simulink model "sampleModel2072_pp"  (R2021a)
settings: Solver=VariableStepAuto  StartTime=0.0  StopTime=10.0  RelTol=1e-3
undefined symbols (not defined in the file or in its folder): DiscIntNeverNeededParam, magnitude, Newton, Raphson
libraries: simulink x184, pid_lib x33
(part 3 of 5)

== system sampleModel2072_pp/cfblk39/cfblk6 ==
  cfblk1 : Inport
  cfblk10 : Signum
  cfblk11 : Sin  TimeSource=Use external signal  SampleTime=0
  cfblk12 : Product  Inputs=**
  cfblk13 : Product
  cfblk14 : Delay  SampleTime=1
  cfblk3 : pid_lib/PID Controller  Controller=PID  Form=Parallel  TimeDomain=Discrete-time  UseExternalTs=off  SampleTime=1  IntegratorMethod=Forward Euler  FilterMethod=Forward Euler  ControllerParametersSource=internal  P=1  I=1  D=0  UseFilter=on  N=100  TunerSelectOption=Transfer Function Based (PID Tuner App)  InitialConditionSource=internal  InitialConditionForIntegrator=0  InitialConditionForFilter=0  DifferentiatorICPrevScaledInput=0  ExternalReset=none  TrackingMode=off  Kt=1  LimitOutput=off  SatLimitsSource=internal  UpperSaturationLimit=inf  LowerSaturationLimit=-inf  LinearizeAsGain=off  AntiWindupMode=none  Kb=1  POutMin=[]  POutMax=[]  IOutMin=[]  IOutMax=[]  DOutMin=[]  DOutMax=[]  NOutMin=[]  NOutMax=[]  SumOutMin=[]  SumOutMax=[]  SaturationOutMin=[]  SaturationOutMax=[]  PParamMin=[]  PParamMax=[]  IParamMin=[]  IParamMax=[]  DParamMin=[]  DParamMax=[]  NParamMin=[]  NParamMax=[]  KbParamMin=[]  KbParamMax=[]  KtParamMin=[]  KtParamMax=[]  KbOutMin=[]  KbOutMax=[]  KtOutMin=[]  KtOutMax=[]  IntegratorOutMin=[]  IntegratorOutMax=[]  FilterOutMin=[]  FilterOutMax=[]  SumI1OutMin=[]  SumI1OutMax=[]  SumI2OutMin=[]  SumI2OutMax=[]  SumI3OutMin=[]  SumI3OutMax=[]  SumI4OutMin=[]  SumI4OutMax=[]  SumDOutMin=[]  SumDOutMax=[]  DifferentiatorOutMin=[]  DifferentiatorOutMax=[]  FilterDiffOutCoefMin=[]  FilterDiffOutCoefMax=[]  ReciprocalOutMin=[]  ReciprocalOutMax=[]  SumDenOutMin=[]  SumDenOutMax=[]  SumNumOutMin=[]  SumNumOutMax=[]  DivideOutMin=[]  DivideOutMax=[]  UdiffTsProdOutMin=[]  UdiffTsProdOutMax=[]  NTsProdOutMin=[]  NTsProdOutMax=[]  UintegralTsProdOutMin=[]  UintegralTsProdOutMax=[]  UngainTsProdOutMin=[]  UngainTsProdOutMax=[]  IntegratorContinuousStateAttributes=''  IntegratorStateMustResolveToSignalObject=off  IntegratorRTWStateStorageClass=Auto  FilterContinuousStateAttributes=''  FilterStateMustResolveToSignalObject=off  FilterRTWStateStorageClass=Auto  ParallelPVariant=InternalParameters  IdealPVariant=Disabled  IVariant=InternalParameters  DVariant=InternalParameters  IntegratorVariant=Discrete  SatVariant=Disabled  AWVariant=Passthrough  PCopyVariant=Disabled  TRVariant=Disabled  FdbkBlocksVariant=Forward  IdealPFdbkVariant=Disabled  SatFdbkVariant=Disabled  DerivativeFilterVariant=ForwardEulerFilter  NVariant=InternalParameters  NCopyVariant=Disabled  FilterICVariant=InternalICsFilter  IntegratorICVariant=InternalICs  ExternalResetVariant=Disabled  TRSumVariant=Passthrough  SumFdbkVariant=Disabled  SumVariant=Sum_PID  TsampFilterVariant=InternalTs  TsampNgainVariant=Passthrough  TsampIntegralVariant=Passthrough  ExternalSaturationOutDataTypeStr=Inherit: Same as second input
  cfblk4 : simulink/Discrete/Transfer Fcn Lead or Lag  PoleZ=0.95  ZeroZ=0.75  ICPrevOutput=0.0  ICPrevInput=0.0  DoSatur=off
      settings: SourceProductBaseCode=SL
  cfblk5 : Product  Inputs=**
  cfblk6 : Sqrt  Operator=rSqrt  AlgorithmType=Newton-Raphson  SaturateOnIntegerOverflow=on
  cfblk7 : Sqrt  SaturateOnIntegerOverflow=on
  cfblk8 : Gain  Gain=[-748975620.675067]
  cfblk9 : Reshape
  cfblk2 : Outport
  wires:
  cfblk5/1 -> cfblk3/1
  cfblk7/1 -> cfblk10/1
  cfblk4/1 -> cfblk7/1
  cfblk3/1 -> cfblk6/1
  cfblk1/1 -> cfblk9/1
  cfblk12/1 -> cfblk11/1
  cfblk10/1 -> cfblk13/1, cfblk12/1
  cfblk6/1 -> cfblk8/1
  cfblk9/1 -> cfblk4/1
  cfblk11/1 -> cfblk2/1
  cfblk13/1 -> cfblk5/1, cfblk5/2, cfblk12/2
  cfblk8/1 -> cfblk14/1
  cfblk14/1 -> cfblk13/2

== system sampleModel2072_pp/cfblk39/cfblk7 ==
  cfblk1 : Inport
  cfblk3 : simulink/Discrete/Transfer Fcn First Order  PoleZ=0.95  ICPrevOutput=0.0  DoSatur=off
  cfblk4 : Sqrt  SaturateOnIntegerOverflow=on
  cfblk5 : Product  Inputs=**
  cfblk6 : Gain  Gain=[-247254324.663936]
  cfblk7 : Sqrt  SaturateOnIntegerOverflow=on
  cfblk8 : Polyval  Coefs=[ +2.081618890e-019, -1.441693666e-014, +4.719686976e-010, -8.536869453e-006, +1.621573104e-001, -8.087801117e+001 ]
  cfblk9 : Delay  SampleTime=1
  cfblk2 : Outport
  wires:
  cfblk3/1 -> cfblk8/1
  cfblk7/1 -> cfblk3/1
  cfblk6/1 -> cfblk4/1
  cfblk4/1 -> cfblk2/1
  cfblk5/1 -> cfblk7/1
  cfblk1/1 -> cfblk6/1, cfblk5/2
  cfblk8/1 -> cfblk9/1
  cfblk9/1 -> cfblk5/1

== system sampleModel2072_pp/cfblk39/cfblk8 ==
  cfblk1 : Inport
  cfblk10 : Gain  Gain=[-609988645.580152]
  cfblk11 : Sqrt  SaturateOnIntegerOverflow=on
  cfblk12 : Rounding
  cfblk13 : Reshape
  cfblk14 : Delay  SampleTime=1
  cfblk15 : Delay  SampleTime=1
  cfblk3 : DiscreteZeroPole  Poles=[0 0.5]  Gain=1
  cfblk4 : DiscreteIntegrator  ICPrevOutput=DiscIntNeverNeededParam  ICPrevScaledInput=DiscIntNeverNeededParam
  cfblk5 : simulink/Discrete/Tapped Delay  vinit=0.0  samptime=-1  NumDelays=1  DelayOrder=Oldest  includeCurrent=off
  cfblk6 : Sum  Inputs=|++
  cfblk7 : Rounding
  cfblk8 : Product
  cfblk9 : Math  Operator=log  SaturateOnIntegerOverflow=on
  cfblk2 : Outport
  wires:
  cfblk8/1 -> cfblk9/1
  cfblk4/1 -> cfblk11/1
  cfblk12/1 -> cfblk2/1, cfblk13/1
  cfblk6/1 -> cfblk3/1
  cfblk3/1 -> cfblk8/1
  cfblk10/1 -> cfblk4/1
  cfblk5/1 -> cfblk6/1
  cfblk11/1 -> cfblk7/1
  cfblk1/1 -> cfblk6/2, cfblk10/1
  cfblk7/1 -> cfblk5/1
  cfblk9/1 -> cfblk14/1
  cfblk14/1 -> cfblk8/2
  cfblk13/1 -> cfblk15/1
  cfblk15/1 -> cfblk12/1

== system sampleModel2072_pp/cfblk40/cfblk10 ==
  cfblk1 : Inport
  cfblk8 : Inport  Port=2
  cfblk3 : simulink/Discrete/Transfer Fcn First Order  PoleZ=0.95  ICPrevOutput=0.0  DoSatur=off
  cfblk4 : simulink/Discrete/Transfer Fcn Lead or Lag  PoleZ=0.95  ZeroZ=0.75  ICPrevOutput=0.0  ICPrevInput=0.0  DoSatur=off
      settings: SourceProductBaseCode=SL
  cfblk5 : Rounding
  cfblk6 : Sum
  cfblk7 : MinMax  Function=max
  cfblk2 : Outport
  wires:
  cfblk7/1 -> cfblk5/1
  cfblk1/1 -> cfblk4/1
  cfblk8/1 -> cfblk7/1
  cfblk4/1 -> cfblk6/1
  cfblk5/1 -> cfblk3/1
  cfblk3/1 -> cfblk6/2
  cfblk6/1 -> cfblk2/1

== system sampleModel2072_pp/cfblk40/cfblk11 ==
  cfblk1 : Inport
  cfblk10 : Sum  Inputs=+-
  cfblk11 : Sqrt  SaturateOnIntegerOverflow=on
  cfblk12 : Abs
  cfblk13 : Sum  Inputs=+
  cfblk14 : Product  Inputs=**
  cfblk15 : MinMax  Function=max  Inputs=3
  cfblk16 : Delay  SampleTime=1
  cfblk17 : Delay  SampleTime=1
  cfblk18 : Delay  SampleTime=1
  cfblk3 : simulink/Discrete/Transfer Fcn Real Zero  ZeroZ=0.75  ICPrevInput=0.0  DoSatur=off
      settings: SourceProductBaseCode=SL
  cfblk4 : MinMax  Function=max  Inputs=2
  cfblk5 : PermuteDimensions
  cfblk6 : Trigonometry
  cfblk7 : Signum
  cfblk8 : Sqrt  SaturateOnIntegerOverflow=on
  cfblk9 : Gain  Gain=[-702374637.657523]
  cfblk2 : Outport
  wires:
  cfblk3/1 -> cfblk8/1
  cfblk6/1 -> cfblk10/1, cfblk7/1
  cfblk13/1 -> cfblk3/1
  cfblk1/1 -> cfblk11/1
  cfblk14/1 -> cfblk15/1
  cfblk12/1 -> cfblk6/1, cfblk15/3, cfblk9/1
  cfblk11/1 -> cfblk4/1, cfblk13/1
  cfblk9/1 -> cfblk15/2, cfblk2/1
  cfblk4/1 -> cfblk10/2
  cfblk5/1 -> cfblk12/1
  cfblk8/1 -> cfblk14/2
  cfblk10/1 -> cfblk16/1
  cfblk16/1 -> cfblk4/2
  cfblk15/1 -> cfblk17/1
  cfblk17/1 -> cfblk14/1
  cfblk7/1 -> cfblk18/1
  cfblk18/1 -> cfblk5/1

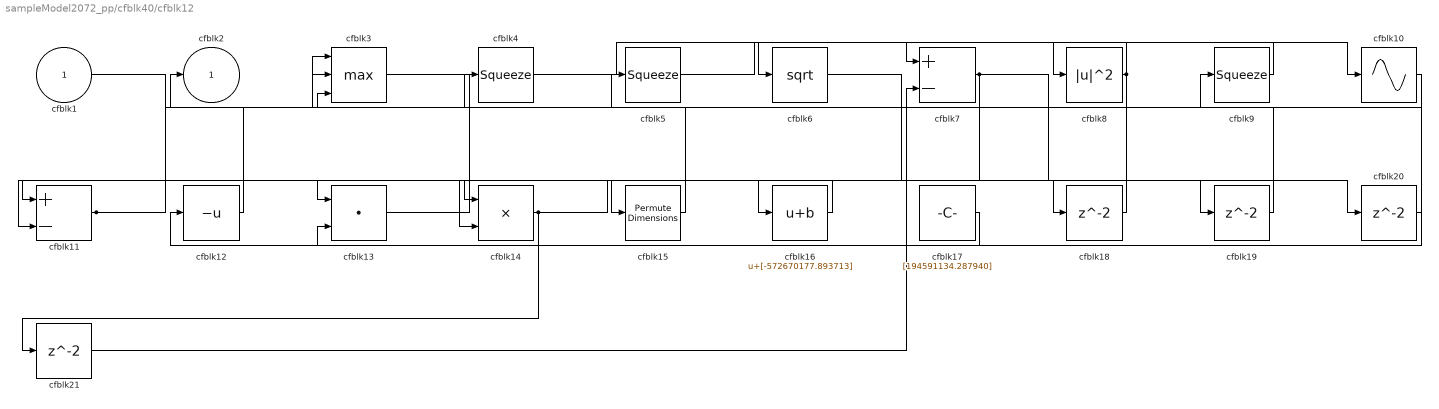
== system sampleModel2072_pp/cfblk40/cfblk12 ==
  cfblk1 : Inport
  cfblk10 : Sin  TimeSource=Use external signal  SampleTime=0
  cfblk11 : Sum  Inputs=+-
  cfblk12 : UnaryMinus
  cfblk13 : DotProduct  InputSameDT=on  OutDataTypeStr=Inherit: Inherit via internal rule
  cfblk14 : Product  Inputs=**
  cfblk15 : PermuteDimensions
  cfblk16 : Bias  Bias=[-572670177.893713]
  cfblk17 : Constant  Value=[194591134.287940]  SampleTime=1
  cfblk{18..21} (4 alike) : Delay  SampleTime=1
  cfblk3 : MinMax  Function=max  Inputs=3
  cfblk4 : Squeeze
  cfblk5 : Squeeze
  cfblk6 : Sqrt  SaturateOnIntegerOverflow=on
  cfblk7 : Sum  Inputs=+-
  cfblk8 : Math  Operator=magnitude^2  SaturateOnIntegerOverflow=on
  cfblk9 : Squeeze
  cfblk2 : Outport
  wires:
  cfblk4/1 -> cfblk10/1
  cfblk3/1 -> cfblk16/1
  cfblk7/1 -> cfblk14/2, cfblk19/1
  cfblk10/1 -> cfblk12/1
  cfblk14/1 -> cfblk20/1, cfblk21/1
  cfblk11/1 -> cfblk5/1, cfblk14/1
  cfblk13/1 -> cfblk9/1
  cfblk9/1 -> cfblk8/1
  cfblk16/1 -> cfblk13/1
  cfblk12/1 -> cfblk2/1
  cfblk17/1 -> cfblk13/2
  cfblk8/1 -> cfblk6/1, cfblk11/1, cfblk11/2
  cfblk5/1 -> cfblk7/1
  cfblk1/1 -> cfblk15/1
  cfblk15/1 -> cfblk4/1
  cfblk6/1 -> cfblk18/1
  cfblk18/1 -> cfblk3/2
  cfblk19/1 -> cfblk3/1
  cfblk20/1 -> cfblk3/3
  cfblk21/1 -> cfblk7/2

== system sampleModel2072_pp/cfblk41/cfblk10 ==
  cfblk1 : Inport
  cfblk10 : MinMax  Inputs=3
  cfblk11 : Gain  Gain=[90025695.862637]
  cfblk12 : Product
  cfblk13 : Delay  SampleTime=1
  cfblk3 : Delay  DelayLengthSource=Input port  SampleTime=1
      settings: InputPortMap=u0,p1
  cfblk4 : Rounding
  cfblk5 : ComplexToRealImag
  cfblk6 : Trigonometry
  cfblk7 : MinMax  Function=max
  cfblk8 : Polyval  Coefs=[ +2.081618890e-019, -1.441693666e-014, +4.719686976e-010, -8.536869453e-006, +1.621573104e-001, -8.087801117e+001 ]
  cfblk9 : Product
  cfblk2 : Outport
  wires:
  cfblk1/1 -> cfblk7/1
  cfblk8/1 -> cfblk3/1, cfblk9/2
  cfblk7/1 -> cfblk5/1, cfblk6/1, cfblk9/1
  cfblk9/1 -> cfblk3/2, cfblk12/2
  cfblk3/1 -> cfblk11/1
  cfblk6/1 -> cfblk10/2
  cfblk4/1 -> cfblk10/3
  cfblk10/1 -> cfblk12/1
  cfblk11/1 -> cfblk4/1
  cfblk5/1 -> cfblk2/1
  cfblk5/2 -> cfblk8/1
  cfblk12/1 -> cfblk13/1
  cfblk13/1 -> cfblk10/1

== system sampleModel2072_pp/cfblk41/cfblk11 ==
  cfblk1 : Inport
  cfblk3 : Reshape
  cfblk4 : ComplexToMagnitudeAngle
  cfblk5 : ComplexToRealImag
  cfblk6 : Bias  Bias=[701798241.247478]
  cfblk7 : simulink/Math Operations/Slider Gain  gain=1  low=0  high=2
  cfblk8 : Delay  SampleTime=1
  cfblk2 : Outport
  wires:
  cfblk7/1 -> cfblk3/1
  cfblk3/1 -> cfblk2/1
  cfblk1/1 -> cfblk5/1
  cfblk4/1 -> cfblk7/1
  cfblk4/2 -> cfblk6/1
  cfblk6/1 -> cfblk8/1
  cfblk8/1 -> cfblk4/1

== system sampleModel2072_pp/cfblk41/cfblk7 ==
  cfblk1 : Inport
  cfblk10 : Sum  Inputs=+
  cfblk11 : Rounding
  cfblk12 : Sum  Inputs=|++
  cfblk13 : Product
  cfblk14 : Delay  SampleTime=1
  cfblk3 : Delay  ShowEnablePort=on  SampleTime=1
      settings: InputPortMap=u0,e6
  cfblk4 : DiscreteFilter  SampleTime=1
  cfblk5 : Signum
  cfblk6 : Sin  TimeSource=Use external signal  SampleTime=0
  cfblk7 : Rounding
  cfblk8 : Sum  Inputs=|++
  cfblk9 : simulink/Math Operations/Slider Gain  gain=1  low=0  high=2
  cfblk2 : Outport
  wires:
  cfblk10/1 -> cfblk2/1
  cfblk11/1 -> cfblk6/1
  cfblk13/1 -> cfblk5/1, cfblk14/1
  cfblk1/1 -> cfblk11/1, cfblk13/2
  cfblk12/1 -> cfblk7/1
  cfblk6/1 -> cfblk9/1, cfblk8/1
  cfblk5/1 -> cfblk4/1
  cfblk9/1 -> cfblk3/1, cfblk12/2
  cfblk4/1 -> cfblk3/2
  cfblk3/1 -> cfblk12/1
  cfblk7/1 -> cfblk10/1
  cfblk8/1 -> cfblk13/1
  cfblk14/1 -> cfblk8/2

== system sampleModel2072_pp/cfblk41/cfblk8 ==
  cfblk1 : Inport
  cfblk10 : simulink/Math Operations/Slider Gain  gain=1  low=0  high=2
  cfblk11 : Signum
  cfblk12 : simulink/Math Operations/MinMax Running Resettable  Function=min  vinit=0.0
  cfblk13 : DotProduct  InputSameDT=on  OutDataTypeStr=Inherit: Inherit via internal rule
  cfblk14 : Abs
  cfblk15 : Delay  SampleTime=1
  cfblk3 : simulink/Discrete/Transfer Fcn Lead or Lag  PoleZ=0.95  ZeroZ=0.75  ICPrevOutput=0.0  ICPrevInput=0.0  DoSatur=off
      settings: SourceProductBaseCode=SL
  cfblk4 : DiscreteFilter  SampleTime=1
  cfblk5 : pid_lib/PID Controller  Controller=PID  Form=Parallel  TimeDomain=Discrete-time  UseExternalTs=off  SampleTime=1  IntegratorMethod=Forward Euler  FilterMethod=Forward Euler  ControllerParametersSource=internal  P=1  I=1  D=0  UseFilter=on  N=100  TunerSelectOption=Transfer Function Based (PID Tuner App)  InitialConditionSource=internal  InitialConditionForIntegrator=0  InitialConditionForFilter=0  DifferentiatorICPrevScaledInput=0  ExternalReset=none  TrackingMode=off  Kt=1  LimitOutput=off  SatLimitsSource=internal  UpperSaturationLimit=inf  LowerSaturationLimit=-inf  LinearizeAsGain=off  AntiWindupMode=none  Kb=1  POutMin=[]  POutMax=[]  IOutMin=[]  IOutMax=[]  DOutMin=[]  DOutMax=[]  NOutMin=[]  NOutMax=[]  SumOutMin=[]  SumOutMax=[]  SaturationOutMin=[]  SaturationOutMax=[]  PParamMin=[]  PParamMax=[]  IParamMin=[]  IParamMax=[]  DParamMin=[]  DParamMax=[]  NParamMin=[]  NParamMax=[]  KbParamMin=[]  KbParamMax=[]  KtParamMin=[]  KtParamMax=[]  KbOutMin=[]  KbOutMax=[]  KtOutMin=[]  KtOutMax=[]  IntegratorOutMin=[]  IntegratorOutMax=[]  FilterOutMin=[]  FilterOutMax=[]  SumI1OutMin=[]  SumI1OutMax=[]  SumI2OutMin=[]  SumI2OutMax=[]  SumI3OutMin=[]  SumI3OutMax=[]  SumI4OutMin=[]  SumI4OutMax=[]  SumDOutMin=[]  SumDOutMax=[]  DifferentiatorOutMin=[]  DifferentiatorOutMax=[]  FilterDiffOutCoefMin=[]  FilterDiffOutCoefMax=[]  ReciprocalOutMin=[]  ReciprocalOutMax=[]  SumDenOutMin=[]  SumDenOutMax=[]  SumNumOutMin=[]  SumNumOutMax=[]  DivideOutMin=[]  DivideOutMax=[]  UdiffTsProdOutMin=[]  UdiffTsProdOutMax=[]  NTsProdOutMin=[]  NTsProdOutMax=[]  UintegralTsProdOutMin=[]  UintegralTsProdOutMax=[]  UngainTsProdOutMin=[]  UngainTsProdOutMax=[]  IntegratorContinuousStateAttributes=''  IntegratorStateMustResolveToSignalObject=off  IntegratorRTWStateStorageClass=Auto  FilterContinuousStateAttributes=''  FilterStateMustResolveToSignalObject=off  FilterRTWStateStorageClass=Auto  ParallelPVariant=InternalParameters  IdealPVariant=Disabled  IVariant=InternalParameters  DVariant=InternalParameters  IntegratorVariant=Discrete  SatVariant=Disabled  AWVariant=Passthrough  PCopyVariant=Disabled  TRVariant=Disabled  FdbkBlocksVariant=Forward  IdealPFdbkVariant=Disabled  SatFdbkVariant=Disabled  DerivativeFilterVariant=ForwardEulerFilter  NVariant=InternalParameters  NCopyVariant=Disabled  FilterICVariant=InternalICsFilter  IntegratorICVariant=InternalICs  ExternalResetVariant=Disabled  TRSumVariant=Passthrough  SumFdbkVariant=Disabled  SumVariant=Sum_PID  TsampFilterVariant=InternalTs  TsampNgainVariant=Passthrough  TsampIntegralVariant=Passthrough  ExternalSaturationOutDataTypeStr=Inherit: Same as second input
  cfblk6 : DiscreteZeroPole  Poles=[0 0.5]  Gain=1
  cfblk7 : Sin  TimeSource=Use external signal  SampleTime=0
  cfblk8 : Signum
  cfblk9 : Signum
  cfblk2 : Outport
  wires:
  cfblk8/1 -> cfblk7/1
  cfblk3/1 -> cfblk14/1
  cfblk11/1 -> cfblk6/1, cfblk12/1
  cfblk12/1 -> cfblk2/1
  cfblk6/1 -> cfblk9/1, cfblk12/2
  cfblk4/1 -> cfblk13/1
  cfblk9/1 -> cfblk3/1
  cfblk14/1 -> cfblk4/1
  cfblk1/1 -> cfblk11/1
  cfblk5/1 -> cfblk8/1
  cfblk13/1 -> cfblk10/1
  cfblk10/1 -> cfblk5/1
  cfblk7/1 -> cfblk15/1
  cfblk15/1 -> cfblk13/2

== system sampleModel2072_pp/cfblk41/cfblk9 ==
  cfblk1 : Inport
  cfblk10 : Product
  cfblk11 : ComplexToRealImag
  cfblk12 : Sum  Inputs=-+
  cfblk13 : Assignment  DiagnosticForDimensions=Warning  IndexOptions=Index vector (dialog)  Indices=1  OutputSizes=1
  cfblk14 : Squeeze
  cfblk15 : Product
  cfblk16 : Product  Inputs=*
  cfblk17 : Sqrt  SaturateOnIntegerOverflow=on
  cfblk18 : Delay  SampleTime=1
  cfblk19 : Delay  SampleTime=1
  cfblk3 : pid_lib/PID Controller (2DOF)  Controller=PID  Form=Parallel  TimeDomain=Discrete-time  UseExternalTs=off  SampleTime=1  IntegratorMethod=Forward Euler  FilterMethod=Forward Euler  ControllerParametersSource=internal  P=1  I=1  D=0  UseFilter=on  N=100  b=1  c=1  TunerSelectOption=Transfer Function Based (PID Tuner App)  InitialConditionSource=internal  InitialConditionForIntegrator=0  InitialConditionForFilter=0  DifferentiatorICPrevScaledInput=0  ExternalReset=none  TrackingMode=off  Kt=1  LimitOutput=off  SatLimitsSource=internal  UpperSaturationLimit=inf  LowerSaturationLimit=-inf  LinearizeAsGain=off  AntiWindupMode=none  Kb=1  POutMin=[]  POutMax=[]  IOutMin=[]  IOutMax=[]  DOutMin=[]  DOutMax=[]  NOutMin=[]  NOutMax=[]  bOutMin=[]  bOutMax=[]  cOutMin=[]  cOutMax=[]  SumOutMin=[]  SumOutMax=[]  SaturationOutMin=[]  SaturationOutMax=[]  PParamMin=[]  PParamMax=[]  IParamMin=[]  IParamMax=[]  DParamMin=[]  DParamMax=[]  NParamMin=[]  NParamMax=[]  bParamMin=[]  bParamMax=[]  cParamMin=[]  cParamMax=[]  KbParamMin=[]  KbParamMax=[]  KtParamMin=[]  KtParamMax=[]  KbOutMin=[]  KbOutMax=[]  KtOutMin=[]  KtOutMax=[]  IntegratorOutMin=[]  IntegratorOutMax=[]  FilterOutMin=[]  FilterOutMax=[]  SumI1OutMin=[]  SumI1OutMax=[]  SumI2OutMin=[]  SumI2OutMax=[]  SumI3OutMin=[]  SumI3OutMax=[]  SumI4OutMin=[]  SumI4OutMax=[]  SumDOutMin=[]  SumDOutMax=[]  Sum1OutMin=[]  Sum1OutMax=[]  Sum2OutMin=[]  Sum2OutMax=[]  Sum3OutMin=[]  Sum3OutMax=[]  DifferentiatorOutMin=[]  DifferentiatorOutMax=[]  FilterDiffOutCoefMin=[]  FilterDiffOutCoefMax=[]  ReciprocalOutMin=[]  ReciprocalOutMax=[]  SumDenOutMin=[]  SumDenOutMax=[]  SumNumOutMin=[]  SumNumOutMax=[]  DivideOutMin=[]  DivideOutMax=[]  UdiffTsProdOutMin=[]  UdiffTsProdOutMax=[]  NTsProdOutMin=[]  NTsProdOutMax=[]  UintegralTsProdOutMin=[]  UintegralTsProdOutMax=[]  UngainTsProdOutMin=[]  UngainTsProdOutMax=[]  IntegratorContinuousStateAttributes=''  IntegratorStateMustResolveToSignalObject=off  IntegratorRTWStateStorageClass=Auto  FilterContinuousStateAttributes=''  FilterStateMustResolveToSignalObject=off  FilterRTWStateStorageClass=Auto  ParallelPVariant=InternalParameters  IdealPVariant=Disabled  IVariant=InternalParameters  DVariant=InternalParameters  bVariant=InternalParameters  cVariant=InternalParameters  IntegratorVariant=Discrete  SatVariant=Disabled  AWVariant=Passthrough  PCopyVariant=Disabled  TRVariant=Disabled  FdbkBlocksVariant=Forward  IdealPFdbkVariant=Disabled  SatFdbkVariant=Disabled  DerivativeFilterVariant=ForwardEulerFilter  NVariant=InternalParameters  NCopyVariant=Disabled  FilterICVariant=InternalICsFilter  IntegratorICVariant=InternalICs  ExternalResetVariant=Disabled  TRSumVariant=Passthrough  SumFdbkVariant=Disabled  SumVariant=Sum_PID  TsampFilterVariant=InternalTs  TsampNgainVariant=Passthrough  TsampIntegralVariant=Passthrough  ExternalSaturationOutDataTypeStr=Inherit: Same as second input
      settings: SourceProductBaseCode=SL
  cfblk4 : simulink/Discrete/Transfer Fcn First Order  PoleZ=0.95  ICPrevOutput=0.0  DoSatur=off
  cfblk5 : Delay  SampleTime=1
  cfblk6 : DiscreteStateSpace
  cfblk7 : DotProduct  InputSameDT=on  OutDataTypeStr=Inherit: Inherit via internal rule
  cfblk8 : Reshape
  cfblk9 : Rounding
  cfblk2 : Outport
  wires:
  cfblk15/1 -> cfblk14/1
  cfblk11/1 -> cfblk15/1
  cfblk17/1 -> cfblk6/1
  cfblk3/1 -> cfblk12/1
  cfblk4/1 -> cfblk5/1
  cfblk7/1 -> cfblk9/1
  cfblk10/1 -> cfblk16/1, cfblk19/1
  cfblk1/1 -> cfblk4/1, cfblk10/1
  cfblk5/1 -> cfblk3/1
  cfblk8/1 -> cfblk15/2, cfblk10/2
  cfblk13/1 -> cfblk17/1
  cfblk16/1 -> cfblk13/1
  cfblk11/2 -> cfblk13/2
  cfblk12/1 -> cfblk8/1, cfblk11/1
  cfblk14/1 -> cfblk2/1, cfblk7/2
  cfblk6/1 -> cfblk7/1
  cfblk9/1 -> cfblk18/1
  cfblk18/1 -> cfblk3/2
  cfblk19/1 -> cfblk12/2

== system sampleModel2072_pp/cfblk42/cfblk4 ==
  cfblk1 : Inport
  cfblk10 : Sum  Inputs=|++
  cfblk11 : Trigonometry
  cfblk12 : Polyval  Coefs=[ +2.081618890e-019, -1.441693666e-014, +4.719686976e-010, -8.536869453e-006, +1.621573104e-001, -8.087801117e+001 ]
  cfblk13 : Gain  Gain=[561466155.167679]
  cfblk14 : Assignment  DiagnosticForDimensions=Warning  IndexOptions=Index vector (dialog)  Indices=1  OutputSizes=1
  cfblk15 : Reshape
  cfblk16 : MinMax  Function=max  Inputs=2
  cfblk17 : Delay  SampleTime=1
  cfblk18 : Delay  SampleTime=1
  cfblk19 : Delay  SampleTime=1
  cfblk3 : DiscreteFilter  SampleTime=1
  cfblk4 : simulink/Discrete/Transfer Fcn First Order  PoleZ=0.95  ICPrevOutput=0.0  DoSatur=off
  cfblk5 : simulink/Math Operations/MinMax Running Resettable  Function=min  vinit=0.0
  cfblk6 : Bias  Bias=[572427056.871552]
  cfblk7 : Polyval  Coefs=[ +2.081618890e-019, -1.441693666e-014, +4.719686976e-010, -8.536869453e-006, +1.621573104e-001, -8.087801117e+001 ]
  cfblk8 : simulink/Math Operations/MinMax Running Resettable  Function=min  vinit=0.0
  cfblk9 : Assignment  DiagnosticForDimensions=Warning  IndexOptions=Index vector (dialog)  Indices=1  OutputSizes=1
  cfblk2 : Outport
  wires:
  cfblk16/1 -> cfblk9/1
  cfblk5/1 -> cfblk11/1, cfblk4/1, cfblk19/1
  cfblk14/1 -> cfblk6/1
  cfblk11/1 -> cfblk16/1
  cfblk9/1 -> cfblk8/1
  cfblk3/1 -> cfblk14/1
  cfblk7/1 -> cfblk16/2
  cfblk12/1 -> cfblk8/2
  cfblk10/1 -> cfblk2/1, cfblk13/1
  cfblk6/1 -> cfblk7/1, cfblk15/1, cfblk5/2, cfblk18/1
  cfblk8/1 -> cfblk10/2
  cfblk1/1 -> cfblk12/1
  cfblk4/1 -> cfblk9/2
  cfblk15/1 -> cfblk5/1
  cfblk13/1 -> cfblk17/1
  cfblk17/1 -> cfblk10/1
  cfblk18/1 -> cfblk14/2
  cfblk19/1 -> cfblk3/1

== system sampleModel2072_pp/cfblk42/cfblk5 ==
  cfblk1 : Inport
  cfblk10 : Delay  SampleTime=1
  cfblk3 : DiscreteIntegrator  ICPrevOutput=DiscIntNeverNeededParam  ICPrevScaledInput=DiscIntNeverNeededParam
  cfblk4 : Sum  Inputs=-+
  cfblk5 : Math  Operator=rem  SaturateOnIntegerOverflow=on
  cfblk6 : Sum  Inputs=+
  cfblk7 : Polyval  Coefs=[ +2.081618890e-019, -1.441693666e-014, +4.719686976e-010, -8.536869453e-006, +1.621573104e-001, -8.087801117e+001 ]
  cfblk8 : Sqrt  SaturateOnIntegerOverflow=on
  cfblk9 : Delay  SampleTime=1
  cfblk2 : Outport
  wires:
  cfblk4/1 -> cfblk7/1
  cfblk7/1 -> cfblk6/1
  cfblk6/1 -> cfblk5/1, cfblk10/1
  cfblk3/1 -> cfblk2/1
  cfblk5/1 -> cfblk8/1, cfblk3/1
  cfblk1/1 -> cfblk4/1
  cfblk8/1 -> cfblk9/1
  cfblk9/1 -> cfblk5/2
  cfblk10/1 -> cfblk4/2

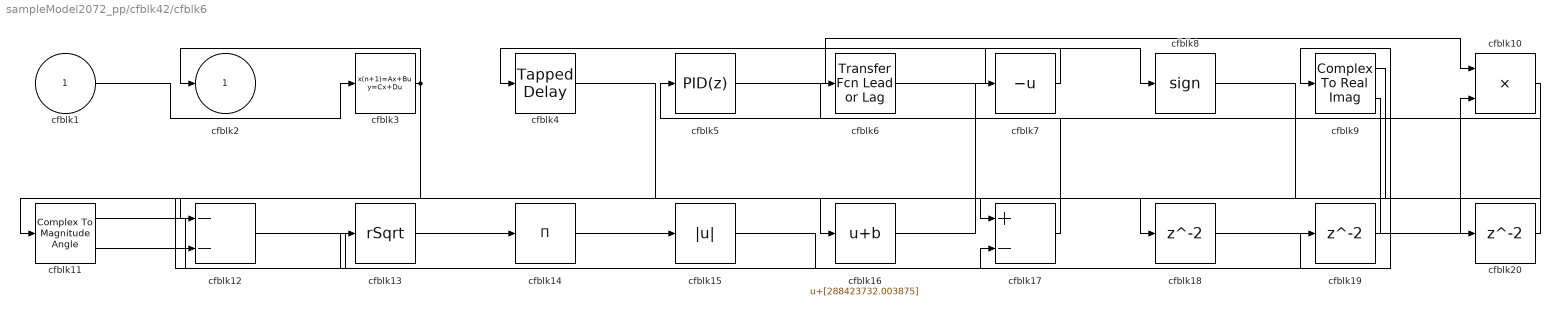
== system sampleModel2072_pp/cfblk42/cfblk6 ==
  cfblk1 : Inport
  cfblk10 : Product  Inputs=**
  cfblk11 : ComplexToMagnitudeAngle
  cfblk12 : Sum  Inputs=--
  cfblk13 : Sqrt  Operator=rSqrt  AlgorithmType=Newton-Raphson  SaturateOnIntegerOverflow=on
  cfblk14 : Product  Inputs=*
  cfblk15 : Abs
  cfblk16 : Bias  Bias=[288423732.003875]
  cfblk17 : Sum  Inputs=+-
  cfblk18 : Delay  SampleTime=1
  cfblk19 : Delay  SampleTime=1
  cfblk20 : Delay  SampleTime=1
  cfblk3 : DiscreteStateSpace
  cfblk4 : simulink/Discrete/Tapped Delay  vinit=0.0  samptime=-1  NumDelays=1  DelayOrder=Oldest  includeCurrent=off
  cfblk5 : pid_lib/PID Controller  Controller=PID  Form=Parallel  TimeDomain=Discrete-time  UseExternalTs=off  SampleTime=1  IntegratorMethod=Forward Euler  FilterMethod=Forward Euler  ControllerParametersSource=internal  P=1  I=1  D=0  UseFilter=on  N=100  TunerSelectOption=Transfer Function Based (PID Tuner App)  InitialConditionSource=internal  InitialConditionForIntegrator=0  InitialConditionForFilter=0  DifferentiatorICPrevScaledInput=0  ExternalReset=none  TrackingMode=off  Kt=1  LimitOutput=off  SatLimitsSource=internal  UpperSaturationLimit=inf  LowerSaturationLimit=-inf  LinearizeAsGain=off  AntiWindupMode=none  Kb=1  POutMin=[]  POutMax=[]  IOutMin=[]  IOutMax=[]  DOutMin=[]  DOutMax=[]  NOutMin=[]  NOutMax=[]  SumOutMin=[]  SumOutMax=[]  SaturationOutMin=[]  SaturationOutMax=[]  PParamMin=[]  PParamMax=[]  IParamMin=[]  IParamMax=[]  DParamMin=[]  DParamMax=[]  NParamMin=[]  NParamMax=[]  KbParamMin=[]  KbParamMax=[]  KtParamMin=[]  KtParamMax=[]  KbOutMin=[]  KbOutMax=[]  KtOutMin=[]  KtOutMax=[]  IntegratorOutMin=[]  IntegratorOutMax=[]  FilterOutMin=[]  FilterOutMax=[]  SumI1OutMin=[]  SumI1OutMax=[]  SumI2OutMin=[]  SumI2OutMax=[]  SumI3OutMin=[]  SumI3OutMax=[]  SumI4OutMin=[]  SumI4OutMax=[]  SumDOutMin=[]  SumDOutMax=[]  DifferentiatorOutMin=[]  DifferentiatorOutMax=[]  FilterDiffOutCoefMin=[]  FilterDiffOutCoefMax=[]  ReciprocalOutMin=[]  ReciprocalOutMax=[]  SumDenOutMin=[]  SumDenOutMax=[]  SumNumOutMin=[]  SumNumOutMax=[]  DivideOutMin=[]  DivideOutMax=[]  UdiffTsProdOutMin=[]  UdiffTsProdOutMax=[]  NTsProdOutMin=[]  NTsProdOutMax=[]  UintegralTsProdOutMin=[]  UintegralTsProdOutMax=[]  UngainTsProdOutMin=[]  UngainTsProdOutMax=[]  IntegratorContinuousStateAttributes=''  IntegratorStateMustResolveToSignalObject=off  IntegratorRTWStateStorageClass=Auto  FilterContinuousStateAttributes=''  FilterStateMustResolveToSignalObject=off  FilterRTWStateStorageClass=Auto  ParallelPVariant=InternalParameters  IdealPVariant=Disabled  IVariant=InternalParameters  DVariant=InternalParameters  IntegratorVariant=Discrete  SatVariant=Disabled  AWVariant=Passthrough  PCopyVariant=Disabled  TRVariant=Disabled  FdbkBlocksVariant=Forward  IdealPFdbkVariant=Disabled  SatFdbkVariant=Disabled  DerivativeFilterVariant=ForwardEulerFilter  NVariant=InternalParameters  NCopyVariant=Disabled  FilterICVariant=InternalICsFilter  IntegratorICVariant=InternalICs  ExternalResetVariant=Disabled  TRSumVariant=Passthrough  SumFdbkVariant=Disabled  SumVariant=Sum_PID  TsampFilterVariant=InternalTs  TsampNgainVariant=Passthrough  TsampIntegralVariant=Passthrough  ExternalSaturationOutDataTypeStr=Inherit: Same as second input
  cfblk6 : simulink/Discrete/Transfer Fcn Lead or Lag  PoleZ=0.95  ZeroZ=0.75  ICPrevOutput=0.0  ICPrevInput=0.0  DoSatur=off
      settings: SourceProductBaseCode=SL
  cfblk7 : UnaryMinus
  cfblk8 : Signum
  cfblk9 : ComplexToRealImag
  cfblk2 : Outport
  wires:
  cfblk9/1 -> cfblk11/1
  cfblk12/1 -> cfblk9/1
  cfblk13/1 -> cfblk14/1
  cfblk10/1 -> cfblk16/1
  cfblk3/1 -> cfblk2/1, cfblk12/2
  cfblk11/1 -> cfblk13/1
  cfblk6/1 -> cfblk8/1
  cfblk9/2 -> cfblk17/1
  cfblk17/1 -> cfblk5/1
  cfblk5/1 -> cfblk10/1
  cfblk7/1 -> cfblk4/1
  cfblk16/1 -> cfblk7/1
  cfblk14/1 -> cfblk15/1
  cfblk1/1 -> cfblk3/1
  cfblk15/1 -> cfblk17/2
  cfblk4/1 -> cfblk18/1
  cfblk18/1 -> cfblk10/2
  cfblk11/2 -> cfblk19/1
  cfblk19/1 -> cfblk12/1
  cfblk8/1 -> cfblk20/1
  cfblk20/1 -> cfblk6/1

== system sampleModel2072_pp/cfblk42/cfblk7 ==
  cfblk1 : Inport
  cfblk3 : simulink/Discrete/Difference  ICPrevInput=0.0  OutMin=[]  OutMax=[]  OutDataTypeStr=Inherit: Inherit via back propagation  OutDataType=fixdt(1, 16)  OutScaling=2^-10  DoSatur=off
  cfblk4 : DiscreteFir  SampleTime=1
  cfblk5 : Delay  ShowEnablePort=on  SampleTime=1
      settings: InputPortMap=u0,e6
  cfblk6 : DotProduct  InputSameDT=on  OutDataTypeStr=Inherit: Inherit via internal rule
  cfblk7 : Squeeze
  cfblk8 : Delay  SampleTime=1
  cfblk2 : Outport
  wires:
  cfblk4/1 -> cfblk3/1
  cfblk1/1 -> cfblk5/1
  cfblk3/1 -> cfblk7/1
  cfblk7/1 -> cfblk2/1, cfblk6/2
  cfblk5/1 -> cfblk4/1, cfblk6/1
  cfblk6/1 -> cfblk8/1
  cfblk8/1 -> cfblk5/2

== system sampleModel2072_pp/cfblk43/cfblk13 ==
  cfblk1 : Inport
  cfblk10 : Delay  SampleTime=1
  cfblk3 : simulink/Discrete/Transfer Fcn First Order  PoleZ=0.95  ICPrevOutput=0.0  DoSatur=off
  cfblk4 : UnitDelay  HasFrameUpgradeWarning=on
  cfblk5 : simulink/Discrete/Tapped Delay  vinit=0.0  samptime=-1  NumDelays=1  DelayOrder=Oldest  includeCurrent=off
  cfblk6 : Signum
  cfblk7 : Sum  Inputs=+
  cfblk8 : Squeeze
  cfblk9 : simulink/Math Operations/Slider Gain  gain=1  low=0  high=2
  cfblk2 : Outport
  wires:
  cfblk3/1 -> cfblk4/1
  cfblk1/1 -> cfblk7/1
  cfblk6/1 -> cfblk9/1
  cfblk5/1 -> cfblk6/1
  cfblk7/1 -> cfblk3/1
  cfblk4/1 -> cfblk2/1, cfblk8/1
  cfblk9/1 -> cfblk10/1
  cfblk10/1 -> cfblk5/1

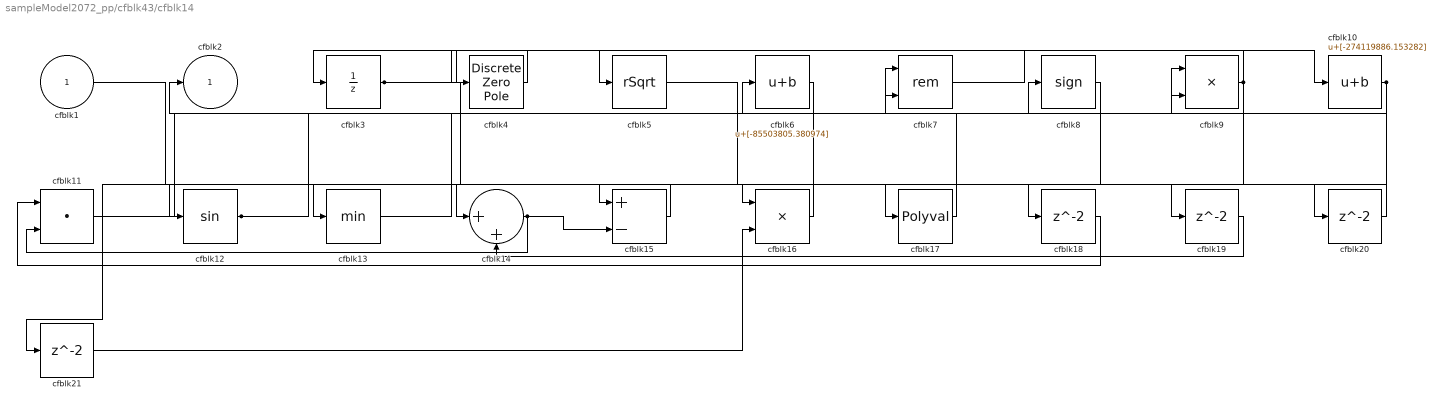
== system sampleModel2072_pp/cfblk43/cfblk14 ==
  cfblk1 : Inport
  cfblk10 : Bias  Bias=[-274119886.153282]
  cfblk11 : DotProduct  InputSameDT=on  OutDataTypeStr=Inherit: Inherit via internal rule
  cfblk12 : Trigonometry
  cfblk13 : MinMax
  cfblk14 : Sum  Inputs=|++
  cfblk15 : Sum  Inputs=+-
  cfblk16 : Product
  cfblk17 : Polyval  Coefs=[ +2.081618890e-019, -1.441693666e-014, +4.719686976e-010, -8.536869453e-006, +1.621573104e-001, -8.087801117e+001 ]
  cfblk{18..21} (4 alike) : Delay  SampleTime=1
  cfblk3 : UnitDelay  HasFrameUpgradeWarning=on
  cfblk4 : DiscreteZeroPole  Poles=[0 0.5]  Gain=1
  cfblk5 : Sqrt  Operator=rSqrt  AlgorithmType=Newton-Raphson  SaturateOnIntegerOverflow=on
  cfblk6 : Bias  Bias=[-85503805.380974]
  cfblk7 : Math  Operator=rem  SaturateOnIntegerOverflow=on
  cfblk8 : Signum
  cfblk9 : Product  Inputs=**
  cfblk2 : Outport
  wires:
  cfblk3/1 -> cfblk17/1, cfblk5/1
  cfblk16/1 -> cfblk6/1
  cfblk4/1 -> cfblk3/1
  cfblk14/1 -> cfblk11/2, cfblk15/2
  cfblk17/1 -> cfblk2/1
  cfblk11/1 -> cfblk7/1
  cfblk6/1 -> cfblk14/1
  cfblk13/1 -> cfblk9/1
  cfblk1/1 -> cfblk16/1
  cfblk15/1 -> cfblk13/1
  cfblk12/1 -> cfblk8/1, cfblk9/2, cfblk19/1
  cfblk9/1 -> cfblk4/1, cfblk21/1
  cfblk7/1 -> cfblk10/1
  cfblk10/1 -> cfblk12/1, cfblk15/1
  cfblk8/1 -> cfblk18/1
  cfblk18/1 -> cfblk11/1
  cfblk19/1 -> cfblk14/2
  cfblk5/1 -> cfblk20/1
  cfblk20/1 -> cfblk7/2
  cfblk21/1 -> cfblk16/2

== system sampleModel2072_pp/cfblk43/cfblk15 ==
  cfblk1 : Inport
  cfblk11 : Delay  SampleTime=1
  cfblk3 : Delay  DelayLengthSource=Input port  SampleTime=1
      settings: InputPortMap=u0,p1
  cfblk4 : Bias  Bias=[477313716.999227]
  cfblk5 : Product  Inputs=*
  cfblk6 : Assignment  DiagnosticForDimensions=Warning  IndexOptions=Index vector (dialog)  Indices=1  OutputSizes=1
  cfblk7 : simulink/Math Operations/Slider Gain  gain=1  low=0  high=2
  cfblk8 : Product  Inputs=**
  cfblk9 : Constant  Value=[143493398.316818]  SampleTime=1
  cfblk2 : Outport
  cfblk10 : Outport  Port=2
  wires:
  cfblk9/1 -> cfblk6/1, cfblk8/1, cfblk8/2
  cfblk7/1 -> cfblk5/1
  cfblk6/1 -> cfblk2/1
  cfblk3/1 -> cfblk7/1, cfblk6/2
  cfblk8/1 -> cfblk4/1
  cfblk4/1 -> cfblk3/1
  cfblk1/1 -> cfblk10/1
  cfblk5/1 -> cfblk11/1
  cfblk11/1 -> cfblk3/2

== system sampleModel2072_pp/cfblk43/cfblk16 ==
  cfblk1 : Inport
  cfblk3 : simulink/Discrete/Difference  ICPrevInput=0.0  OutMin=[]  OutMax=[]  OutDataTypeStr=Inherit: Inherit via back propagation  OutDataType=fixdt(1, 16)  OutScaling=2^-10  DoSatur=off
  cfblk4 : Abs
  cfblk5 : Sum  Inputs=+-
  cfblk6 : Sqrt  SaturateOnIntegerOverflow=on
  cfblk7 : Abs
  cfblk8 : Gain  Gain=[744900502.933597]
  cfblk9 : Delay  SampleTime=1
  cfblk2 : Outport
  wires:
  cfblk5/1 -> cfblk3/1
  cfblk3/1 -> cfblk4/1
  cfblk6/1 -> cfblk8/1
  cfblk4/1 -> cfblk2/1
  cfblk8/1 -> cfblk5/2, cfblk9/1
  cfblk1/1 -> cfblk7/1
  cfblk7/1 -> cfblk5/1
  cfblk9/1 -> cfblk6/1

== system sampleModel2072_pp/cfblk44/cfblk11 ==
  cfblk1 : Inport
  cfblk10 : Math  SaturateOnIntegerOverflow=on
  cfblk11 : Sum  Inputs=--
  cfblk12 : Sum  Inputs=|++
  cfblk13 : Delay  SampleTime=1
  cfblk14 : Delay  SampleTime=1
  cfblk3 : DiscreteFir  SampleTime=1
  cfblk4 : DiscreteFilter  SampleTime=1
  cfblk5 : Delay  ShowEnablePort=on  SampleTime=1
      settings: InputPortMap=u0,e6
  cfblk6 : Reshape
  cfblk7 : simulink/Math Operations/Slider Gain  gain=1  low=0  high=2
  cfblk8 : Product
  cfblk9 : UnaryMinus
  cfblk2 : Outport
  wires:
  cfblk12/1 -> cfblk6/1, cfblk8/2
  cfblk7/1 -> cfblk11/1, cfblk9/1
  cfblk1/1 -> cfblk7/1
  cfblk11/1 -> cfblk12/1
  cfblk8/1 -> cfblk4/1, cfblk3/1
  cfblk10/1 -> cfblk5/1
  cfblk3/1 -> cfblk2/1
  cfblk6/1 -> cfblk10/1
  cfblk9/1 -> cfblk8/1
  cfblk4/1 -> cfblk5/2, cfblk14/1
  cfblk5/1 -> cfblk13/1
  cfblk13/1 -> cfblk12/2
  cfblk14/1 -> cfblk11/2

== system sampleModel2072_pp/cfblk44/cfblk12 ==
  cfblk1 : Inport
  cfblk10 : Sum  Inputs=|++
  cfblk11 : Product  Inputs=**
  cfblk12 : Math  Operator=log10  SaturateOnIntegerOverflow=on
  cfblk13 : Constant  Value=[366943198.541673]  SampleTime=1
  cfblk14 : Delay  SampleTime=1
  cfblk15 : Delay  SampleTime=1
  cfblk16 : Delay  SampleTime=1
  cfblk3 : simulink/Discrete/Tapped Delay  vinit=0.0  samptime=-1  NumDelays=1  DelayOrder=Oldest  includeCurrent=off
  cfblk4 : DiscreteZeroPole  Poles=[0 0.5]  Gain=1
  cfblk5 : Rounding
  cfblk6 : Sum
  cfblk7 : Assignment  DiagnosticForDimensions=Warning  IndexOptions=Index vector (dialog)  Indices=1  OutputSizes=1
  cfblk8 : Math  Operator=hermitian  SaturateOnIntegerOverflow=on
  cfblk9 : Assignment  DiagnosticForDimensions=Warning  IndexOptions=Index vector (dialog)  Indices=1  OutputSizes=1
  cfblk2 : Outport
  wires:
  cfblk6/1 -> cfblk7/2
  cfblk9/1 -> cfblk8/1
  cfblk8/1 -> cfblk5/1
  cfblk13/1 -> cfblk11/1
  cfblk5/1 -> cfblk4/1, cfblk10/2
  cfblk4/1 -> cfblk2/1, cfblk16/1
  cfblk3/1 -> cfblk11/2, cfblk14/1
  cfblk7/1 -> cfblk10/1
  cfblk1/1 -> cfblk12/1, cfblk9/2
  cfblk12/1 -> cfblk6/2
  cfblk10/1 -> cfblk3/1
  cfblk14/1 -> cfblk6/1
  cfblk11/1 -> cfblk15/1
  cfblk15/1 -> cfblk7/1
  cfblk16/1 -> cfblk9/1

== system sampleModel2072_pp/cfblk44/cfblk14 ==
  cfblk1 : Inport
  Action Port : ActionPort  ActionPortLabel=if(u1 >= 0)
  cfblk3 : simulink/Discrete/Transfer Fcn Lead or Lag  PoleZ=0.95  ZeroZ=0.75  ICPrevOutput=0.0  ICPrevInput=0.0  DoSatur=off
      settings: SourceProductBaseCode=SL
  cfblk4 : DiscreteZeroPole  Poles=[0 0.5]  Gain=1  SampleTime=-1
  cfblk5 : Reshape
  cfblk6 : Polyval  Coefs=[ +2.081618890e-019, -1.441693666e-014, +4.719686976e-010, -8.536869453e-006, +1.621573104e-001, -8.087801117e+001 ]
  cfblk7 : Math  Operator=hypot  SaturateOnIntegerOverflow=on
  cfblk8 : UnaryMinus
  cfblk9 : Delay
  cfblk2 : Outport
  wires:
  cfblk7/1 -> cfblk2/1
  cfblk8/1 -> cfblk6/1
  cfblk3/1 -> cfblk7/1
  cfblk1/1 -> cfblk3/1
  cfblk5/1 -> cfblk8/1, cfblk4/1
  cfblk4/1 -> cfblk7/2
  cfblk6/1 -> cfblk9/1
  cfblk9/1 -> cfblk5/1

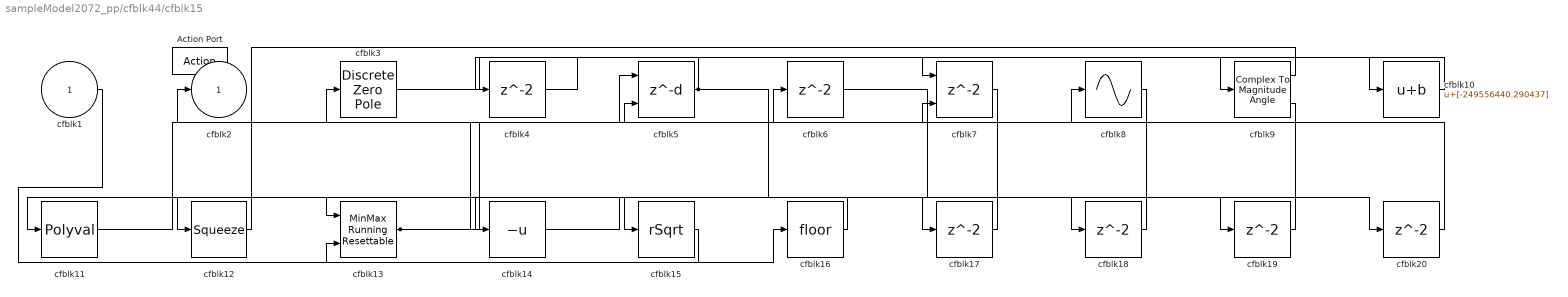
== system sampleModel2072_pp/cfblk44/cfblk15 ==
  cfblk1 : Inport
  Action Port : ActionPort  ActionPortLabel=else
  cfblk10 : Bias  Bias=[-249556440.290437]
  cfblk11 : Polyval  Coefs=[ +2.081618890e-019, -1.441693666e-014, +4.719686976e-010, -8.536869453e-006, +1.621573104e-001, -8.087801117e+001 ]
  cfblk12 : Squeeze
  cfblk13 : simulink/Math Operations/MinMax Running Resettable  Function=min  vinit=0.0
  cfblk14 : UnaryMinus
  cfblk15 : Sqrt  Operator=rSqrt  AlgorithmType=Newton-Raphson  SaturateOnIntegerOverflow=on
  cfblk16 : Rounding
  cfblk{4,6,17..20} (6 alike) : Delay
  cfblk3 : DiscreteZeroPole  Poles=[0 0.5]  Gain=1  SampleTime=-1
  cfblk5 : Delay  DelayLengthSource=Input port
      settings: InputPortMap=u0,p1
  cfblk7 : Delay  ShowEnablePort=on
      settings: InputPortMap=u0,e6
  cfblk8 : Sin  TimeSource=Use external signal  SampleTime=0
  cfblk9 : ComplexToMagnitudeAngle
  cfblk2 : Outport
  wires:
  cfblk4/1 -> cfblk9/1
  cfblk9/1 -> cfblk11/1
  cfblk1/1 -> cfblk16/1
  cfblk13/1 -> cfblk5/2, cfblk6/1
  cfblk16/1 -> cfblk12/1
  cfblk3/1 -> cfblk10/1
  cfblk10/1 -> cfblk7/1
  cfblk12/1 -> cfblk2/1
  cfblk5/1 -> cfblk4/1, cfblk17/1
  cfblk15/1 -> cfblk13/2
  cfblk7/1 -> cfblk15/1
  cfblk11/1 -> cfblk8/1
  cfblk9/2 -> cfblk14/1
  cfblk17/1 -> cfblk3/1
  cfblk8/1 -> cfblk18/1
  cfblk18/1 -> cfblk13/1
  cfblk14/1 -> cfblk19/1
  cfblk19/1 -> cfblk5/1
  cfblk6/1 -> cfblk20/1
  cfblk20/1 -> cfblk7/2

== system sampleModel2072_pp/cfblk45/cfblk12 ==
  cfblk1 : Inport
  cfblk3 : DiscreteStateSpace
  cfblk4 : Math  Operator=conj  SaturateOnIntegerOverflow=on
  cfblk5 : Squeeze
  cfblk6 : Sin  TimeSource=Use external signal  SampleTime=0
  cfblk7 : Sum
  cfblk8 : Reshape
  cfblk9 : Delay  SampleTime=1
  cfblk2 : Outport
  wires:
  cfblk1/1 -> cfblk7/1
  cfblk4/1 -> cfblk2/1
  cfblk8/1 -> cfblk5/1
  cfblk6/1 -> cfblk4/1, cfblk3/1
  cfblk7/1 -> cfblk8/1
  cfblk5/1 -> cfblk6/1
  cfblk3/1 -> cfblk9/1
  cfblk9/1 -> cfblk7/2

== system sampleModel2072_pp/cfblk45/cfblk13 ==
  cfblk1 : Inport
  cfblk10 : Product  Inputs=**
  cfblk11 : Sum  Inputs=+
  cfblk12 : DotProduct  InputSameDT=on  OutDataTypeStr=Inherit: Inherit via internal rule
  cfblk13 : PermuteDimensions
  cfblk14 : Product
  cfblk15 : Sin  TimeSource=Use external signal  SampleTime=0
  cfblk16 : Delay  SampleTime=1
  cfblk17 : Delay  SampleTime=1
  cfblk3 : DiscreteZeroPole  Poles=[0 0.5]  Gain=1
  cfblk4 : simulink/Discrete/Difference  ICPrevInput=0.0  OutMin=[]  OutMax=[]  OutDataTypeStr=Inherit: Inherit via back propagation  OutDataType=fixdt(1, 16)  OutScaling=2^-10  DoSatur=off
  cfblk5 : UnitDelay  HasFrameUpgradeWarning=on
  cfblk6 : simulink/Math Operations/Slider Gain  gain=1  low=0  high=2
  cfblk7 : Bias  Bias=[628525833.351052]
  cfblk8 : Polyval  Coefs=[ +2.081618890e-019, -1.441693666e-014, +4.719686976e-010, -8.536869453e-006, +1.621573104e-001, -8.087801117e+001 ]
  cfblk9 : Sum  Inputs=|++
  cfblk2 : Outport
  wires:
  cfblk4/1 -> cfblk2/1, cfblk17/1
  cfblk1/1 -> cfblk10/1
  cfblk12/1 -> cfblk7/1
  cfblk14/1 -> cfblk4/1
  cfblk15/1 -> cfblk8/1
  cfblk7/1 -> cfblk11/1
  cfblk9/1 -> cfblk6/1
  cfblk10/1 -> cfblk9/2, cfblk12/2, cfblk14/2
  cfblk6/1 -> cfblk3/1
  cfblk3/1 -> cfblk5/1, cfblk14/1
  cfblk13/1 -> cfblk15/1
  cfblk5/1 -> cfblk13/1
  cfblk8/1 -> cfblk12/1
  cfblk11/1 -> cfblk16/1
  cfblk16/1 -> cfblk10/2
  cfblk17/1 -> cfblk9/1

== system sampleModel2072_pp/cfblk46/cfblk10 ==
  cfblk1 : Inport
  cfblk10 : Bias  Bias=[-186915168.068286]
  cfblk11 : Delay  SampleTime=1
  cfblk3 : simulink/Discrete/Transfer Fcn Real Zero  ZeroZ=0.75  ICPrevInput=0.0  DoSatur=off
      settings: SourceProductBaseCode=SL
  cfblk4 : DiscreteFir  SampleTime=1
  cfblk5 : Signum
  cfblk6 : Squeeze
  cfblk7 : Sin  TimeSource=Use external signal  SampleTime=0
  cfblk8 : Gain  Gain=[-464886100.243916]
  cfblk9 : Polyval  Coefs=[ +2.081618890e-019, -1.441693666e-014, +4.719686976e-010, -8.536869453e-006, +1.621573104e-001, -8.087801117e+001 ]
  cfblk2 : Outport
  wires:
  cfblk4/1 -> cfblk6/1
  cfblk3/1 -> cfblk10/1
  cfblk5/1 -> cfblk3/1
  cfblk10/1 -> cfblk2/1
  cfblk7/1 -> cfblk5/1
  cfblk9/1 -> cfblk7/1
  cfblk1/1 -> cfblk9/1
  cfblk6/1 -> cfblk8/1
  cfblk8/1 -> cfblk11/1
  cfblk11/1 -> cfblk4/1

== system sampleModel2072_pp/cfblk46/cfblk11 ==
  cfblk1 : Inport
  cfblk3 : pid_lib/PID Controller (2DOF)  Controller=PID  Form=Parallel  TimeDomain=Discrete-time  UseExternalTs=off  SampleTime=1  IntegratorMethod=Forward Euler  FilterMethod=Forward Euler  ControllerParametersSource=internal  P=1  I=1  D=0  UseFilter=on  N=100  b=1  c=1  TunerSelectOption=Transfer Function Based (PID Tuner App)  InitialConditionSource=internal  InitialConditionForIntegrator=0  InitialConditionForFilter=0  DifferentiatorICPrevScaledInput=0  ExternalReset=none  TrackingMode=off  Kt=1  LimitOutput=off  SatLimitsSource=internal  UpperSaturationLimit=inf  LowerSaturationLimit=-inf  LinearizeAsGain=off  AntiWindupMode=none  Kb=1  POutMin=[]  POutMax=[]  IOutMin=[]  IOutMax=[]  DOutMin=[]  DOutMax=[]  NOutMin=[]  NOutMax=[]  bOutMin=[]  bOutMax=[]  cOutMin=[]  cOutMax=[]  SumOutMin=[]  SumOutMax=[]  SaturationOutMin=[]  SaturationOutMax=[]  PParamMin=[]  PParamMax=[]  IParamMin=[]  IParamMax=[]  DParamMin=[]  DParamMax=[]  NParamMin=[]  NParamMax=[]  bParamMin=[]  bParamMax=[]  cParamMin=[]  cParamMax=[]  KbParamMin=[]  KbParamMax=[]  KtParamMin=[]  KtParamMax=[]  KbOutMin=[]  KbOutMax=[]  KtOutMin=[]  KtOutMax=[]  IntegratorOutMin=[]  IntegratorOutMax=[]  FilterOutMin=[]  FilterOutMax=[]  SumI1OutMin=[]  SumI1OutMax=[]  SumI2OutMin=[]  SumI2OutMax=[]  SumI3OutMin=[]  SumI3OutMax=[]  SumI4OutMin=[]  SumI4OutMax=[]  SumDOutMin=[]  SumDOutMax=[]  Sum1OutMin=[]  Sum1OutMax=[]  Sum2OutMin=[]  Sum2OutMax=[]  Sum3OutMin=[]  Sum3OutMax=[]  DifferentiatorOutMin=[]  DifferentiatorOutMax=[]  FilterDiffOutCoefMin=[]  FilterDiffOutCoefMax=[]  ReciprocalOutMin=[]  ReciprocalOutMax=[]  SumDenOutMin=[]  SumDenOutMax=[]  SumNumOutMin=[]  SumNumOutMax=[]  DivideOutMin=[]  DivideOutMax=[]  UdiffTsProdOutMin=[]  UdiffTsProdOutMax=[]  NTsProdOutMin=[]  NTsProdOutMax=[]  UintegralTsProdOutMin=[]  UintegralTsProdOutMax=[]  UngainTsProdOutMin=[]  UngainTsProdOutMax=[]  IntegratorContinuousStateAttributes=''  IntegratorStateMustResolveToSignalObject=off  IntegratorRTWStateStorageClass=Auto  FilterContinuousStateAttributes=''  FilterStateMustResolveToSignalObject=off  FilterRTWStateStorageClass=Auto  ParallelPVariant=InternalParameters  IdealPVariant=Disabled  IVariant=InternalParameters  DVariant=InternalParameters  bVariant=InternalParameters  cVariant=InternalParameters  IntegratorVariant=Discrete  SatVariant=Disabled  AWVariant=Passthrough  PCopyVariant=Disabled  TRVariant=Disabled  FdbkBlocksVariant=Forward  IdealPFdbkVariant=Disabled  SatFdbkVariant=Disabled  DerivativeFilterVariant=ForwardEulerFilter  NVariant=InternalParameters  NCopyVariant=Disabled  FilterICVariant=InternalICsFilter  IntegratorICVariant=InternalICs  ExternalResetVariant=Disabled  TRSumVariant=Passthrough  SumFdbkVariant=Disabled  SumVariant=Sum_PID  TsampFilterVariant=InternalTs  TsampNgainVariant=Passthrough  TsampIntegralVariant=Passthrough  ExternalSaturationOutDataTypeStr=Inherit: Same as second input
      settings: SourceProductBaseCode=SL
  cfblk4 : simulink/Discrete/Transfer Fcn First Order  PoleZ=0.95  ICPrevOutput=0.0  DoSatur=off
  cfblk5 : Delay  SampleTime=1
  cfblk6 : Signum
  cfblk7 : Trigonometry
  cfblk8 : Delay  SampleTime=1
  cfblk2 : Outport
  wires:
  cfblk3/1 -> cfblk4/1
  cfblk5/1 -> cfblk6/1
  cfblk7/1 -> cfblk5/1
  cfblk1/1 -> cfblk3/2
  cfblk4/1 -> cfblk2/1, cfblk7/1
  cfblk6/1 -> cfblk8/1
  cfblk8/1 -> cfblk3/1

== system sampleModel2072_pp/cfblk46/cfblk12 ==
  cfblk1 : Inport
  cfblk10 : Delay  SampleTime=1
  cfblk3 : Signum
  cfblk4 : Product  Inputs=*
  cfblk5 : MinMax  Function=max  Inputs=2
  cfblk6 : Bias  Bias=[601401732.595949]
  cfblk7 : simulink/Math Operations/Slider Gain  gain=1  low=0  high=2
  cfblk8 : Trigonometry
  cfblk9 : Product  Inputs=**
  cfblk2 : Outport
  wires:
  cfblk7/1 -> cfblk8/1, cfblk9/1
  cfblk5/1 -> cfblk7/1
  cfblk8/1 -> cfblk4/1, cfblk9/2
  cfblk4/1 -> cfblk2/1
  cfblk1/1 -> cfblk6/1
  cfblk3/1 -> cfblk5/2
  cfblk6/1 -> cfblk3/1
  cfblk9/1 -> cfblk10/1
  cfblk10/1 -> cfblk5/1

== system sampleModel2072_pp/cfblk46/cfblk9 ==
  cfblk1 : Inport
  cfblk10 : Sum
  cfblk11 : PermuteDimensions
  cfblk12 : Delay  SampleTime=1
  cfblk13 : Delay  SampleTime=1
  cfblk14 : Delay  SampleTime=1
  cfblk3 : simulink/Discrete/Tapped Delay  vinit=0.0  samptime=-1  NumDelays=1  DelayOrder=Oldest  includeCurrent=off
  cfblk4 : simulink/Discrete/Transfer Fcn Real Zero  ZeroZ=0.75  ICPrevInput=0.0  DoSatur=off
      settings: SourceProductBaseCode=SL
  cfblk5 : simulink/Discrete/Transfer Fcn First Order  PoleZ=0.95  ICPrevOutput=0.0  DoSatur=off
  cfblk6 : Sum  Inputs=-+
  cfblk7 : Product
  cfblk8 : Sum  Inputs=+-
  cfblk9 : ComplexToMagnitudeAngle
  cfblk2 : Outport
  wires:
  cfblk5/1 -> cfblk7/1
  cfblk1/1 -> cfblk5/1
  cfblk10/1 -> cfblk11/1
  cfblk9/2 -> cfblk6/2, cfblk13/1
  cfblk8/1 -> cfblk4/1
  cfblk7/1 -> cfblk10/2
  cfblk4/1 -> cfblk2/1, cfblk3/1
  cfblk11/1 -> cfblk9/1
  cfblk6/1 -> cfblk8/1, cfblk8/2
  cfblk9/1 -> cfblk12/1
  cfblk12/1 -> cfblk10/1
  cfblk13/1 -> cfblk7/2
  cfblk3/1 -> cfblk14/1
  cfblk14/1 -> cfblk6/1

== system sampleModel2072_pp/cfblk47/cfblk13 ==
  cfblk1 : Inport
  cfblk10 : Delay  SampleTime=1
  cfblk3 : simulink/Discrete/Transfer Fcn Real Zero  ZeroZ=0.75  ICPrevInput=0.0  DoSatur=off
      settings: SourceProductBaseCode=SL
  cfblk4 : simulink/Discrete/Transfer Fcn First Order  PoleZ=0.95  ICPrevOutput=0.0  DoSatur=off
  cfblk5 : DiscreteFir  SampleTime=1
  cfblk6 : simulink/Discrete/Transfer Fcn Lead or Lag  PoleZ=0.95  ZeroZ=0.75  ICPrevOutput=0.0  ICPrevInput=0.0  DoSatur=off
      settings: SourceProductBaseCode=SL
  cfblk7 : Product  Inputs=*
  cfblk8 : UnaryMinus
  cfblk9 : Delay  SampleTime=1
  cfblk2 : Outport
  wires:
  cfblk1/1 -> cfblk7/1
  cfblk8/1 -> cfblk6/1
  cfblk4/1 -> cfblk5/1
  cfblk7/1 -> cfblk2/1
  cfblk3/1 -> cfblk8/1
  cfblk6/1 -> cfblk9/1
  cfblk9/1 -> cfblk3/1
  cfblk5/1 -> cfblk10/1
  cfblk10/1 -> cfblk4/1

== system sampleModel2072_pp/cfblk49/cfblk12 ==
  cfblk1 : Inport
  cfblk3 : pid_lib/PID Controller  Controller=PID  Form=Parallel  TimeDomain=Discrete-time  UseExternalTs=off  SampleTime=1  IntegratorMethod=Forward Euler  FilterMethod=Forward Euler  ControllerParametersSource=internal  P=1  I=1  D=0  UseFilter=on  N=100  TunerSelectOption=Transfer Function Based (PID Tuner App)  InitialConditionSource=internal  InitialConditionForIntegrator=0  InitialConditionForFilter=0  DifferentiatorICPrevScaledInput=0  ExternalReset=none  TrackingMode=off  Kt=1  LimitOutput=off  SatLimitsSource=internal  UpperSaturationLimit=inf  LowerSaturationLimit=-inf  LinearizeAsGain=off  AntiWindupMode=none  Kb=1  POutMin=[]  POutMax=[]  IOutMin=[]  IOutMax=[]  DOutMin=[]  DOutMax=[]  NOutMin=[]  NOutMax=[]  SumOutMin=[]  SumOutMax=[]  SaturationOutMin=[]  SaturationOutMax=[]  PParamMin=[]  PParamMax=[]  IParamMin=[]  IParamMax=[]  DParamMin=[]  DParamMax=[]  NParamMin=[]  NParamMax=[]  KbParamMin=[]  KbParamMax=[]  KtParamMin=[]  KtParamMax=[]  KbOutMin=[]  KbOutMax=[]  KtOutMin=[]  KtOutMax=[]  IntegratorOutMin=[]  IntegratorOutMax=[]  FilterOutMin=[]  FilterOutMax=[]  SumI1OutMin=[]  SumI1OutMax=[]  SumI2OutMin=[]  SumI2OutMax=[]  SumI3OutMin=[]  SumI3OutMax=[]  SumI4OutMin=[]  SumI4OutMax=[]  SumDOutMin=[]  SumDOutMax=[]  DifferentiatorOutMin=[]  DifferentiatorOutMax=[]  FilterDiffOutCoefMin=[]  FilterDiffOutCoefMax=[]  ReciprocalOutMin=[]  ReciprocalOutMax=[]  SumDenOutMin=[]  SumDenOutMax=[]  SumNumOutMin=[]  SumNumOutMax=[]  DivideOutMin=[]  DivideOutMax=[]  UdiffTsProdOutMin=[]  UdiffTsProdOutMax=[]  NTsProdOutMin=[]  NTsProdOutMax=[]  UintegralTsProdOutMin=[]  UintegralTsProdOutMax=[]  UngainTsProdOutMin=[]  UngainTsProdOutMax=[]  IntegratorContinuousStateAttributes=''  IntegratorStateMustResolveToSignalObject=off  IntegratorRTWStateStorageClass=Auto  FilterContinuousStateAttributes=''  FilterStateMustResolveToSignalObject=off  FilterRTWStateStorageClass=Auto  ParallelPVariant=InternalParameters  IdealPVariant=Disabled  IVariant=InternalParameters  DVariant=InternalParameters  IntegratorVariant=Discrete  SatVariant=Disabled  AWVariant=Passthrough  PCopyVariant=Disabled  TRVariant=Disabled  FdbkBlocksVariant=Forward  IdealPFdbkVariant=Disabled  SatFdbkVariant=Disabled  DerivativeFilterVariant=ForwardEulerFilter  NVariant=InternalParameters  NCopyVariant=Disabled  FilterICVariant=InternalICsFilter  IntegratorICVariant=InternalICs  ExternalResetVariant=Disabled  TRSumVariant=Passthrough  SumFdbkVariant=Disabled  SumVariant=Sum_PID  TsampFilterVariant=InternalTs  TsampNgainVariant=Passthrough  TsampIntegralVariant=Passthrough  ExternalSaturationOutDataTypeStr=Inherit: Same as second input
  cfblk4 : simulink/Discrete/Transfer Fcn Lead or Lag  PoleZ=0.95  ZeroZ=0.75  ICPrevOutput=0.0  ICPrevInput=0.0  DoSatur=off
      settings: SourceProductBaseCode=SL
  cfblk5 : Abs
  cfblk6 : Math  Operator=mod  SaturateOnIntegerOverflow=on
  cfblk7 : Squeeze
  cfblk8 : Delay  SampleTime=1
  cfblk2 : Outport
  wires:
  cfblk6/1 -> cfblk3/1
  cfblk5/1 -> cfblk2/1
  cfblk3/1 -> cfblk7/1
  cfblk7/1 -> cfblk4/1, cfblk5/1
  cfblk1/1 -> cfblk6/2
  cfblk4/1 -> cfblk8/1
  cfblk8/1 -> cfblk6/1

== system sampleModel2072_pp/cfblk49/cfblk13 ==
  cfblk1 : Inport
  cfblk3 : DiscreteTransferFcn  SampleTime=1
  cfblk4 : simulink/Discrete/Difference  ICPrevInput=0.0  OutMin=[]  OutMax=[]  OutDataTypeStr=Inherit: Inherit via back propagation  OutDataType=fixdt(1, 16)  OutScaling=2^-10  DoSatur=off
  cfblk5 : Polyval  Coefs=[ +2.081618890e-019, -1.441693666e-014, +4.719686976e-010, -8.536869453e-006, +1.621573104e-001, -8.087801117e+001 ]
  cfblk6 : Product  Inputs=**
  cfblk7 : MinMax
  cfblk8 : Sin  TimeSource=Use external signal  SampleTime=0
  cfblk9 : Constant  Value=[-889653633.727904]  SampleTime=1
  cfblk2 : Outport
  wires:
  cfblk1/1 -> cfblk6/1
  cfblk9/1 -> cfblk3/1
  cfblk7/1 -> cfblk6/2
  cfblk6/1 -> cfblk2/1
  cfblk8/1 -> cfblk7/1
  cfblk3/1 -> cfblk5/1, cfblk4/1
  cfblk5/1 -> cfblk8/1
